simulink model "CheckMate_clipboard"  (R2013a)
settings: Solver=ode45  StartTime=0.0  StopTime=200  RelTol=1e-3
PreLoadFcn:
  | acc_setup
libraries: cmlib x7, simulink x1
settings Model: Creator=Zhan  LastModifiedBy=zhan
settings SolverCC: InsertRTBMode=Auto
settings DataIOCC: SignalLoggingSaveFormat=ModelDataLogs  SignalLoggingName=sigsOut
settings OptimizationCC: BooleanDataType=off  ExpressionDepthLimit=2147483647  InitFltsAndDblsToZero=on
settings DebuggingCC: SaveWithParameterizedLinksMsg=none  SignalResolutionControl=TryResolveAllWithWarning  SolverPrmCheckMsg=none  MultiTaskDSMMsg=warning  MultiTaskCondExecSysMsg=none  FcnCallInpInsideContextMsg=UseLocalSettings  StrictBusMsg=None
settings HardwareCC: TargetUnknown=on
settings SFSimCC: SimParseCustomCode=off
settings RTWCC: IncludeERTFirstTime=on
settings GRTTargetCC: CombineOutputUpdateFcns=off  GRTInterface=on

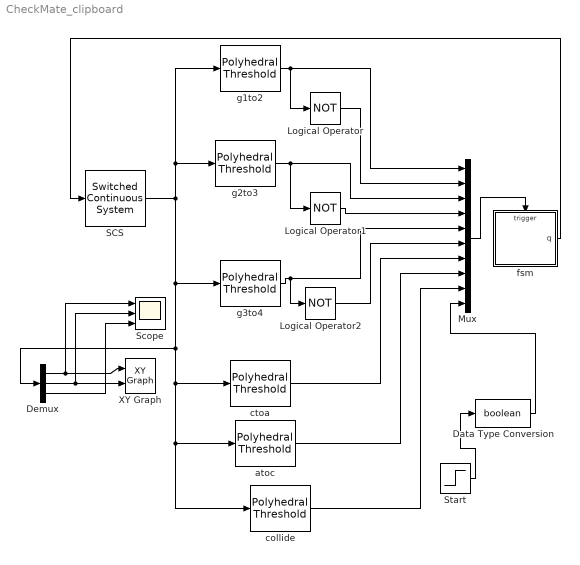
== system CheckMate_clipboard ==
  Data Type Conversion : DataTypeConversion  OutDataTypeStr=boolean  SaturateOnIntegerOverflow=on  RndMeth=Zero
  Demux : Demux  Outputs=3
  Logical Operator : Logic  Operator=NOT
  Logical Operator1 : Logic  Operator=NOT
  Logical Operator2 : Logic  Operator=NOT
  Mux : Mux  Inputs=10
  SCS : cmlib/Switched Continuous System  nx=3  use_sd=off  nup=[]  nz=[]  use_reset=off  nu=1  x0=[40; 1; 0.101]  swfunc=acc_dyn  ICS=Initial_Set  AR=Analysis_Region  use_param=off  p0=[]  PaCs=[]
  Scope : Scope  NumInputPorts=3
      settings: YMin=42~24.4~-75  YMax=42.8~26~375
  Start : Step  Time=0.001  SampleTime=0
  XY Graph : simulink/Sinks/XY Graph  xmin=0  xmax=400  ymin=0  ymax=45  st=-1
  atoc : cmlib/Polyhedral Threshold  polyhedron=tocc
  collide : cmlib/Polyhedral Threshold  polyhedron=collide
  ctoa : cmlib/Polyhedral Threshold  polyhedron=toacc
  fsm : Stateflow chart  TreatAsAtomicUnit=on
  g1to2 : cmlib/Polyhedral Threshold  polyhedron=gear1to2
  g2to3 : cmlib/Polyhedral Threshold  polyhedron=gear2to3
  g3to4 : cmlib/Polyhedral Threshold  polyhedron=gear3to4
  wires:
  SCS/1 -> g3to4/1, ctoa/1, collide/1, atoc/1, Demux/1, g1to2/1, g2to3/1
  g1to2/1 -> Logical Operator/1, Mux/1
  Logical Operator/1 -> Mux/2
  g2to3/1 -> Mux/3, Logical Operator1/1
  Logical Operator1/1 -> Mux/4
  g3to4/1 -> Mux/5, Logical Operator2/1
  Logical Operator2/1 -> Mux/6
  ctoa/1 -> Mux/7
  fsm/1(q) -> SCS/1
  collide/1 -> Mux/9
  Mux/1 -> fsm/Trigger
  atoc/1 -> Mux/8
  Demux/1 -> XY Graph/1, Scope/1
  Demux/2 -> XY Graph/2, Scope/2
  Start/1 -> Data Type Conversion/1
  Data Type Conversion/1 -> Mux/10
  Demux/3 -> Scope/3

== stateflow chart CheckMate_clipboard/fsm ==
  state ACC_1/
    q=5;
  state CC_1/
    q=1;
  state CC_2/
    q=2;
  state ACC_2/
    q=6;
  state avoid_error/
    q=9;
  state CC_3/
    q=3;
  state ACC_3/
    q=7;
  state ACC_4/
    q=8;
  state CC_4/
    q=4;
  CC_1 -> ACC_1 [order 1] : cc_to_acc
  ACC_1 -> avoid_error [order 1] : collide
  (default) -> CC_1 : start
  ACC_1 -> CC_1 [order 3] : acc_to_cc
  ACC_2 -> ACC_1 [order 1] : gear2to1
  ACC_1 -> ACC_2 [order 2] : gear1to2
  CC_2 -> CC_1 [order 1] : gear2to1
  CC_1 -> CC_2 [order 2] : gear1to2
  CC_2 -> ACC_2 [order 2] : cc_to_acc
  ACC_2 -> avoid_error [order 2] : collide
  ACC_2 -> CC_2 [order 4] : acc_to_cc
  CC_3 -> CC_2 [order 1] : gear3to2
  CC_2 -> CC_3 [order 3] : gear2to3
  ACC_3 -> ACC_2 [order 1] : gear3to2
  ACC_2 -> ACC_3 [order 3] : gear2to3
  ACC_3 -> avoid_error [order 2] : collide
  ACC_4 -> avoid_error [order 2] : collide
  CC_3 -> ACC_3 [order 2] : cc_to_acc
  ACC_3 -> CC_3 [order 4] : acc_to_cc
  CC_4 -> CC_3 [order 1] : gear4to3
  CC_3 -> CC_4 [order 3] : gear3to4
  ACC_4 -> ACC_3 [order 1] : gear4to3
  ACC_3 -> ACC_4 [order 3] : gear3to4
  CC_4 -> ACC_4 [order 2] : cc_to_acc
  ACC_4 -> CC_4 [order 3] : acc_to_cc
  data: q output int8
  events: gear1to2 input RISING_EDGE_EVENT; gear2to1 input RISING_EDGE_EVENT; gear2to3 input RISING_EDGE_EVENT; gear3to2 input RISING_EDGE_EVENT; gear3to4 input RISING_EDGE_EVENT; gear4to3 input RISING_EDGE_EVENT; cc_to_acc input RISING_EDGE_EVENT; acc_to_cc input RISING_EDGE_EVENT; collide input RISING_EDGE_EVENT; start input RISING_EDGE_EVENT
